simulink model "simuLab2"  (R2023b)
settings: Solver=VariableStepAuto  StartTime=0.0  StopTime=50  RelTol=1e-3
libraries: simulink_extras x2
settings Model: Creator=tonir  LastModifiedBy=tonir

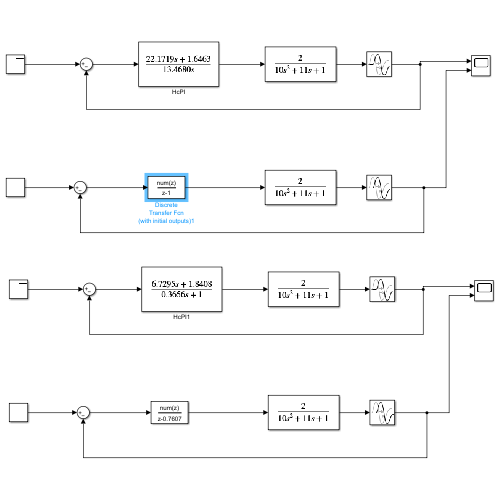
[thumbnail: Simulink's stored preview of the top-level diagram]
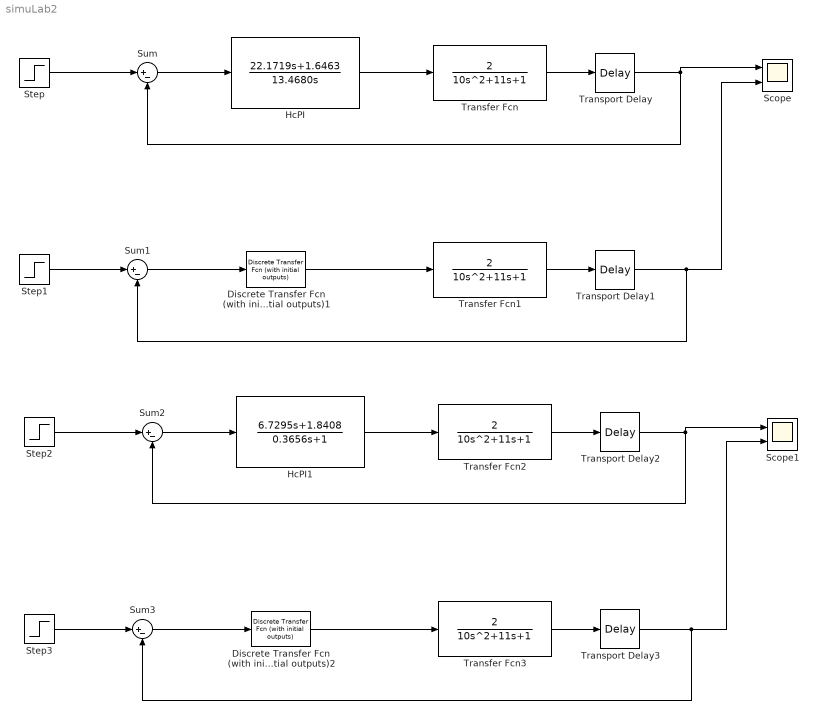
== system simuLab2 ==
  Discrete Transfer Fcn (with initial outputs)1 : simulink_extras/Additional Discrete/Discrete Transfer Fcn (with initial outputs)  N=[1.6463 -1.6340]  D=[1 -1]  U0=0  Y0=0  TS=0.1
  Discrete Transfer Fcn (with initial outputs)2 : simulink_extras/Additional Discrete/Discrete Transfer Fcn (with initial outputs)  N=[18.4077 -17.9672]  D=[1 -0.7607]  U0=0  Y0=0  TS=0.1
  HcPI : TransferFcn  Numerator=[22.1719 1.6463]  Denominator=[13.4680 0]
  HcPI1 : TransferFcn  Numerator=[6.7295 1.8408]  Denominator=[0.3656 1]
  Scope : Scope  NumInputPorts=2
  Scope1 : Scope  NumInputPorts=2
  Step{,1..3} (4 alike) : Step  SampleTime=0
  Sum{,1..3} (4 alike) : Sum  Inputs=|+-
  Transfer Fcn{,1..3} (4 alike) : TransferFcn  Numerator=[2]  Denominator=[10 11 1]
  Transport Delay{,1..3} (4 alike) : TransportDelay
  wires:
  Step/1 -> Sum/1
  Step1/1 -> Sum1/1
  Transport Delay/1 -> Scope/1, Sum/2
  Transport Delay1/1 -> Scope/2, Sum1/2
  Sum/1 -> HcPI/1
  HcPI/1 -> Transfer Fcn/1
  Transfer Fcn/1 -> Transport Delay/1
  Sum1/1 -> Discrete Transfer Fcn (with initial outputs)1/1
  Discrete Transfer Fcn (with initial outputs)1/1 -> Transfer Fcn1/1
  Transfer Fcn1/1 -> Transport Delay1/1
  Discrete Transfer Fcn (with initial outputs)2/1 -> Transfer Fcn3/1
  Transfer Fcn3/1 -> Transport Delay3/1
  Sum2/1 -> HcPI1/1
  HcPI1/1 -> Transfer Fcn2/1
  Transport Delay3/1 -> Scope1/2, Sum3/2
  Transfer Fcn2/1 -> Transport Delay2/1
  Transport Delay2/1 -> Scope1/1, Sum2/2
  Step3/1 -> Sum3/1
  Step2/1 -> Sum2/1
  Sum3/1 -> Discrete Transfer Fcn (with initial outputs)2/1
